simulink model "20240109_HVDCMMCInterconnection"  (R2023b)
settings: Solver=FixedStepDiscrete  StartTime=0.0  StopTime=2  FixedStep=Ts_Power  RelTol=1e-4  EnableMultiTasking=on
PreLoadFcn:
  | HVDCMMCInterconnectionParam
StartFcn:
  | tic
StopFcn:
  | toc
values from neighbouring files (symbols this model uses):
  C_PM = 1.758e-3    (= 0.001758)    [HVDCMMCInterconnectionParam.m]
  Cg = 50e-9    (= 5e-08)    [HVDCMMCInterconnectionParam.m]
  D_R = 0.001    [HVDCMMCInterconnectionParam.m]
  D_Rs = 1e8    (= 100000000)    [HVDCMMCInterconnectionParam.m]
  D_Vf = 0    [HVDCMMCInterconnectionParam.m]
  Fnom = 50    [HVDCMMCInterconnectionParam.m]
  HRM = 2    [HVDCMMCInterconnectionParam.m]
  Ki_Ireg = 6    [HVDCMMCInterconnectionParam.m]
  Ki_Preg = 1.0    (= 1)    [HVDCMMCInterconnectionParam.m]
  Ki_Qreg = 1.0    (= 1)    [HVDCMMCInterconnectionParam.m]
  Ki_VDCreg = 100    [HVDCMMCInterconnectionParam.m]
  Kp_Ireg = 0.6    [HVDCMMCInterconnectionParam.m]
  Kp_Preg = 0.5/3    (= 0.166666666667)    [HVDCMMCInterconnectionParam.m]
  Kp_Qreg = 0.5/3    (= 0.166666666667)    [HVDCMMCInterconnectionParam.m]
  Kp_VDCreg = 4    [HVDCMMCInterconnectionParam.m]
  L_cable = 15e-3    (= 0.015)    [HVDCMMCInterconnectionParam.m]
  Larm = Larm_pu*(Zb_ac/(2*pi*Fnom))    [HVDCMMCInterconnectionParam.m]
  Lff = Larm_pu/2    (= 0.075)    [HVDCMMCInterconnectionParam.m]
  Limits_Ireg = [ 2.0  -2.0]    [HVDCMMCInterconnectionParam.m]
  Limits_Preg = [ 1.2, 0.8 ]    [HVDCMMCInterconnectionParam.m]
  Limits_Qreg = [ 0.25, -0.25 ]    [HVDCMMCInterconnectionParam.m]
  Limits_VDCreg = [ 2.0  -2.0]    [HVDCMMCInterconnectionParam.m]
  Lxfo = 0.12    [HVDCMMCInterconnectionParam.m]
  Nb_PM = 36    [HVDCMMCInterconnectionParam.m]
  Pnom = 1000e6    (= 1000000000)    [HVDCMMCInterconnectionParam.m]
  R_cable = 0.5    [HVDCMMCInterconnectionParam.m]
  R_startup = 400    [HVDCMMCInterconnectionParam.m]
  Rarm = Rarm_pu*Zb_ac    [HVDCMMCInterconnectionParam.m]
  Rff = Rarm_pu/2    (= 0.00075)    [HVDCMMCInterconnectionParam.m]
  Rg = 100    [HVDCMMCInterconnectionParam.m]
  Rxfo = 0.003    [HVDCMMCInterconnectionParam.m]
  Slope_Pref = 0.5    [HVDCMMCInterconnectionParam.m]
  Slope_Qref = 0.5    [HVDCMMCInterconnectionParam.m]
  Slope_Vdc_ref = Vnom_dc/5    (= 128000)    [HVDCMMCInterconnectionParam.m]
  Tbrk1_On = 0.1    [HVDCMMCInterconnectionParam.m]
  Tbrk2_On = 1.0    (= 1)    [HVDCMMCInterconnectionParam.m]
  Tdeblock = 1.5    [HVDCMMCInterconnectionParam.m]
  Tfault = 9999    [HVDCMMCInterconnectionParam.m]
  Ton_Converter2 = 4    [HVDCMMCInterconnectionParam.m]
  Ton_PQreg = 4    [HVDCMMCInterconnectionParam.m]
  Ton_VDCreg = 1.5    [HVDCMMCInterconnectionParam.m]
  Ts = Ts_Control    (= 4e-05)    [HVDCMMCInterconnectionParam.m]
  Ts_Control = 40e-6    (= 4e-05)    [HVDCMMCInterconnectionParam.m]
  Ts_Power = 20e-6    (= 2e-05)    [HVDCMMCInterconnectionParam.m]
  Vb_ac = sqrt(2/3)*Vnom_sec    [HVDCMMCInterconnectionParam.m]
  Vb_dc = Vnom_dc    (= 640000)    [HVDCMMCInterconnectionParam.m]
  Vc0_PM = 0    [HVDCMMCInterconnectionParam.m]
  Vnom_dc = 640e3    (= 640000)    [HVDCMMCInterconnectionParam.m]
  Vnom_prim = 400e3    (= 400000)    [HVDCMMCInterconnectionParam.m]
  Vnom_sec = 333e3    (= 333000)    [HVDCMMCInterconnectionParam.m]
  w = 2*pi*Fnom    (= 314.159265359)    [HVDCMMCInterconnectionParam.m]
undefined symbols (not defined in the file or in its folder): DiscIntNeverNeededParam, gcbh, Pcc, S, sps_AC, sps_ACDC2, sps_rtmsupport
libraries: simulink x48, spsControlledVoltageSourceLib x30, spsCurrentMeasurementLib x30, MMC_Lib x30, spsDiodeLib x20, spsSeriesRLCBranchLib x14, powerlib_extras x12, spsVoltageMeasurementLib x12, spsSecondOrderFilterLib x8, spsabctodq0Lib x8, spsGroundLib x7, spsMeanLib x4
(part 1 of 9)
settings Model: SimulationMode=accelerator  Creator=The MathWorks, Inc.  LastModifiedBy=rober
settings SolverCC: ConcurrentTasks=on  ZeroCrossAlgorithm=Adaptive  InsertRTBMode=Always
settings DataIOCC: SaveFormat=StructureWithTime  SaveOutput=off  SignalLogging=off  DSMLogging=off  SaveTime=off  ReturnWorkspaceOutputs=off
settings OptimizationCC: ReuseModelBlockBuffer=off  ExpressionDepthLimit=2147483647  LifeSpan=inf
settings DebuggingCC: UnderspecifiedInitializationDetection=Classic  MergeDetectMultiDrivingBlocksExec=none  SolverPrmCheckMsg=warning  FcnCallInpInsideContextMsg=warning  AllowSymbolicDim=off  StateNameClashWarn=warning  SFUnexpectedBacktrackingDiag=warning  SFNoUnconditionalDefaultTransitionDiag=warning  SFExecutionAtInitializationDiag=none  ArithmeticOperatorsInVariantConditions=warning
settings HardwareCC: ProdBitPerPointer=32  ProdBitPerSizeT=32  ProdBitPerPtrDiffT=32  ProdLargestAtomicFloat=None  ProdIntDivRoundTo=Undefined  ProdEndianess=Unspecified  ProdWordSize=32  ProdHWDeviceType=32-bit Generic
settings ModelReferenceCC: EnableRefExpFcnMdlSchedulingChecks=on  PropagateSignalLabelsOutOfModel=off
settings SFSimCC: SimUseLocalCustomCode=off  CustomCodeUndefinedFunction=UseInterfaceOnly
settings RTWCC: RTWUseLocalCustomCode=off
settings CodeAppCC: StateflowObjectComments=on
settings GRTTargetCC: CombineOutputUpdateFcns=off  GRTInterface=on
settings ConfigComp: CovMetricSettings=dw  CovSaveCumulativeToWorkspaceVar=on  CovSaveSingleToWorkspaceVar=on  CovExternalEMLEnable=off
settings SimscapeCC: SimscapeNormalizeSystem=off

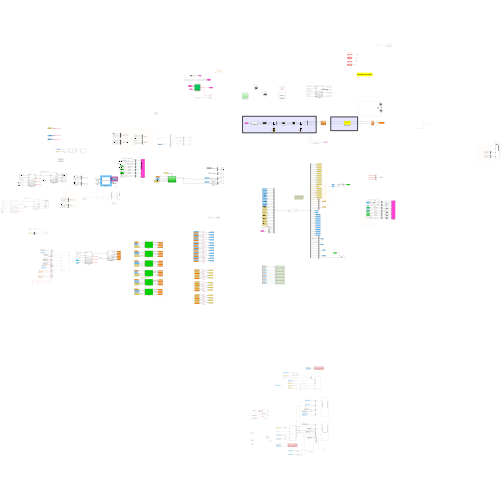
[thumbnail: Simulink's stored preview of the top-level diagram]
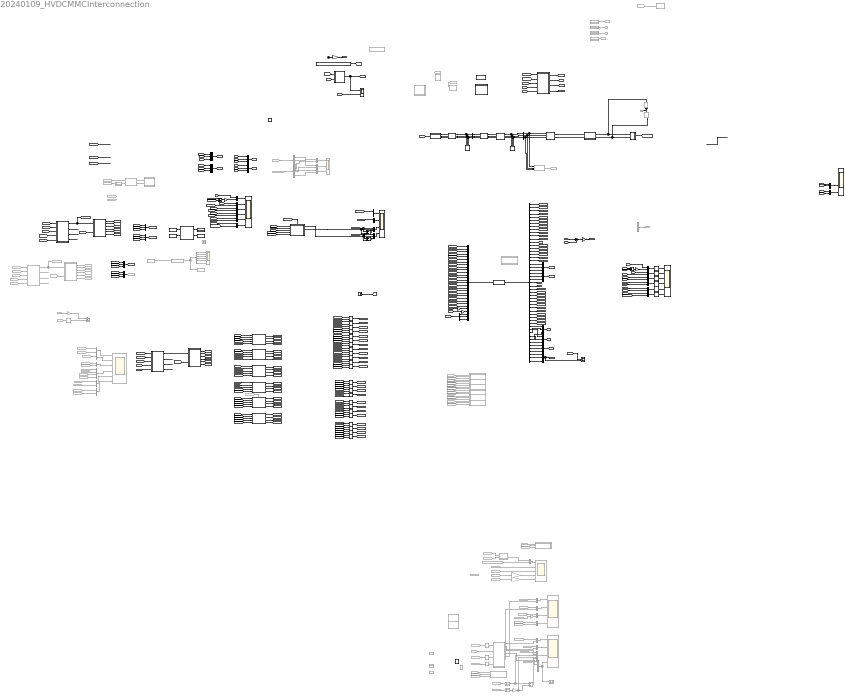
== system 20240109_HVDCMMCInterconnection ==
  note: HVDC-MMC Control System
  3ph SM1 : Subsystem  Commented=on
  3ph SM10 : Subsystem  Commented=on
  3ph SM11 : Subsystem  Commented=on
  3ph SM12 : Subsystem  Commented=on
  3ph SM13 : Subsystem  Commented=on
  3ph SM14 : Subsystem  Commented=on
  3ph SM2 : Subsystem  Commented=on
  3ph SM9 : Subsystem  Commented=on
  Add1 : Sum  Inputs=-+
  Add5 : Sum  Inputs=-+
  Brk1 : spsThreePhaseBreakerLib/Three-Phase Breaker  Commented=on  InitialState=open  SwitchA=on  SwitchB=on  SwitchC=on  SwitchTimes=0.1  External=on  BreakerResistance=0.001  SnubberResistance=1e6  SnubberCapacitance=inf  Measurements=Breaker voltages and currents
  Brk2 : spsThreePhaseBreakerLib/Three-Phase Breaker  Commented=on  InitialState=open  SwitchA=on  SwitchB=on  SwitchC=on  SwitchTimes=[30/60]*10000  External=on  BreakerResistance=0.01  SnubberResistance=1e6  SnubberCapacitance=inf  Measurements=Breaker voltages and currents
  COMPARE : Scope  NumInputPorts=6
  COMPARE1 : Scope  NumInputPorts=6
  Clock : Clock
  Constant3 : Constant  Value=complex( [[ 0 Vnom_prim*sqrt(2/3); 0 0; 0 0] zeros(3,HRM-1) ])
  Control : Subsystem
  Control1 : Subsystem
  Control2 : Subsystem
  Control3 : Subsystem  Commented=on
  Conv 2 : Subsystem
      settings: PortSchema="{\"entries\":[{\"content\":{\"sides\":[{\"content\":{\"connectorIds\":[\"LConn1\",\"LConn2\"]},\"type\":\"ConnectorPlacement.EquallySpacedRectSide\",\"uuid\":\"34e68c3c-08e2-4036-96f4-bd6ca1a4adc7\"},{\"content\":{\"connectorIds\":[\"In1\"],\"side\":\"RIGHT\"},\"type\":\"ConnectorPlacement.EquallySpacedRectSide\",\"uuid\":\"8026f2da-b291-4e86-8efa-4dfa5391ad34\"},{\"content\":{\"side\":\"TOP\"},\"type\":\"ConnectorPlacement.EquallySpacedRectSide\",\"uuid\":\"2a5049d1-3deb-4ece-8237-adb3b31cd77f\"}]},\"type\":\"ConnectorPlacement.EquallySpacedConnector\",\"uuid\":\"95075630-e580-4539-9cf3-c9c75bab0a7f\"}],\"packageUris\":[\"http://schema.mathworks.com/mf0/Connector/R2020b\"],\"version\":\"1.0\"}"
  DC & converter 2 : Subsystem
      mask Display: disp('DC circuit')
  DQn->ABC : MATLAB Function  TreatAsAtomicUnit=on  SystemSampleTime=Ts_Power  mask{N=HRM}
      mask prompts: N "Harmonic order:"
  Delay{,3,10..11} (4 alike) : Delay  Commented=on  DelayLength=1  SampleTime=Ts_Power
  Delay1 : Subsystem  Commented=on
  Delay2 : Delay  DelayLength=1  SampleTime=Ts_Power
  Delay5 : Subsystem  Commented=on
  Delay6 : Subsystem  Commented=on
  Delay7 : Subsystem  Commented=on
  Delay8 : Subsystem  Commented=on
  Delay9 : Subsystem  Commented=on
  Demux : Demux  Outputs=3
  Demux1 : Demux  Commented=on  Outputs=6
  Demux6 : Demux  Outputs=numel(sps_ACDC2.outputs)
  Demux7 : Demux  Commented=on  Outputs=3
  Demux8 : Demux  Commented=on  Outputs=3
  Discrete State-Space : DiscreteStateSpace  A=sps_ACDC2.Adiscrete  B=sps_ACDC2.Bdiscrete  C=sps_ACDC2.Cdiscrete  D=sps_ACDC2.Ddiscrete  InitialCondition=sps_ACDC2.x0  SampleTime=Ts_Power
  Discrete State-Space1 : Subsystem  Commented=on  SystemSampleTime=Ts_Power  mask{A=sps_ACDC2.A, B=sps_ACDC2.B, C=sps_ACDC2.C, D=sps_ACDC2.D, InitVec=sps_ACDC2.x0, dt=Ts_Power, DQSYM=off, N=HRM, Ws=w}
      mask prompts: InitVec "Initial condition:"; dt "Time step (s):"; N "Harmonic number:"; Ws "Angular frequency (1/rad):"
      mask init:
      | % I = eye(size(A,1));
      | % INVR = I/(I-A*dt/2);
      | % Ad1 = INVR*(I+A*dt/2);
      | % Bd1 = INVR*B*dt/2;
      | % Cd1 = C*Ad1;
      | % Dd11 = C*INVR*B*dt/2+D;
      | % Dd12 = C*INVR*B*dt/2;
      | 
      |     I = eye(size(A,1));
      |     INVR = I/(I-A*dt/2);
      |     Ad1 = INVR*(I+A*dt/2);
      |     Bd1 = INVR*B;
      |     Cd1 = C*INVR*dt;
      |     Dd1 = Cd1*B/2 + D;
      | 
      | DQSYM = get_param(gcb,'DQSYM');
      | 
      | comp = 0;
      | 
      | if(strcmp(DQSYM,'on'))
      | 
      | %Calculating the PNZ matrices
      | 
      |     a = -0.5+0.866i;
      |     a2 = -0.5-0.866i;
      |     Sas = [1,a,a2;1,a2,a;1,1,1]/3;
      | 
      |     arows = size(Ad1,1)/3; %signal size
      |     acols = size(Ad1,2)/3; %signal size
      | 
      |     brows = size(Bd1,1)/3; %signal size
      |     bcols = size(Bd1,2)/3; %signal size
      | 
      |     crows = size(Cd1,1)/3; %signal size
      |     ccols = size(Cd1,2)/3; %signal size
      | 
      |     d1rows = size(Dd1,1)/3; %signal size
      |     d1cols = size(Dd1,2)/3; %signal size
      | 
      |     %%%%%%%%%%%%%%%%%%%%%%% Check for inconsistencies  %%%%%%%%%%%%%%%%%%%%%%%
      | 
      |     szMatA = size(A,1);
      |     iL = eye(szMatA);
      |     szMatiL = size(iL,1);
      | 
      |     if(szMatiL ~= szMatA || size(A,1) ~= size(A,2) || size(iL,1) ~= size(iL,2))
      |         error('[Int_DQN_Mat/swFeedback] check matrix A size!');
      |     end
      | 
      |     if(arows ~= brows || acols ~= ccols || crows ~= d1rows || bcols ~= d1cols)
      |         error('[Int_DQN_Mat/Initialize] the sizes of the state-space matrices!');
      |     end
      | 
      |     %%%%%%%%%%%%%%%%%%%%%%%%%%%%%%%%%%%%%%%%%%%%%%%%%%%%%%%%%%%%%%%
      | 
      | 
      |     %%%%%%%%%%%%%%%%%%%%%%% A --> Bpnz %%%%%%%%%%%%%%%%%%%%%%%
      |     Adc = complex(zeros(3*arows,3*acols));
      | 
      |     for i = 1 : arows
      |         for j = 1 : acols
      |             Adc((1:3) + (i-1)*3,(1:3) + (j-1)*3) = Sas*Ad1((1:3) + (i-1)*3,(1:3) + (j-1)*3)/Sas;
      |             %Adc((1:3) + (i-1)*3,(1:3) + (j-1)*3) = diag(diag(real(Adc((1:3) + (i-1)*3,(1:3) + (j-1)*3))));
      |             %Adc((1:3) + (i-1)*3,(1:3) + (j-1)*3) = diag(diag((Adc((1:3) + (i-1)*3,(1:3) + (j-1)*3))));
      | 
      |         end
      |     end
      |     %%%%%%%%%%%%%%%%%%%%%%%%%%%%%%%%%%%%%%%%%%%%%%%%%%%%%%%%%%%%%%%
      | 
      |     %%%%%%%%%%%%%%%%%%%%%%% B --> Bpnz %%%%%%%%%%%%%%%%%%%%%%%
      | 
      |     Bdc = complex(zeros(3*brows,3*bcols));
      | 
      |     for i = 1 : brows
      |         for j = 1 : bcols
      |             Bdc((1:3) + (i-1)*3,(1:3) + (j-1)*3) = Sas*Bd1((1:3) + (i-1)*3,(1:3) + (j-1)*3)/Sas;
      |             %Bdc((1:3) + (i-1)*3,(1:3) + (j-1)*3) = diag(diag(real(Bdc((1:3) + (i-1)*3,(1:3) + (j-1)*3))));
      |             %Bdc((1:3) + (i-1)*3,(1:3) + (j-1)*3) = diag(diag((Bdc((1:3) + (i-1)*3,(1:3) + (j-1)*3))));
      | 
      |         end
      |     end
      |     %%%%%%%%%%%%%%%%%%%%%%%%%%%%%%%%%%%%%%%%%%%%%%%%%%%%%%%%%%%%%%%
      | 
      |     %%%%%%%%%%%%%%%%%%%%%%% C --> Cpnz %%%%%%%%%%%%%%%%%%%%%%%
      | 
      |     Cdc = complex(zeros(3*crows,3*ccols));
      | 
      |     for i = 1 : crows
      |         for j = 1 : ccols
      |             Cdc((1:3) + (i-1)*3,(1:3) + (j-1)*3) = Sas*Cd1((1:3) + (i-1)*3,(1:3) + (j-1)*3)/Sas;
      |             %Cdc((1:3) + (i-1)*3,(1:3) + (j-1)*3) = diag(diag(real(Cdc((1:3) + (i-1)*3,(1:3) + (j-1)*3))));
      |             %Cdc((1:3) + (i-1)*3,(1:3) + (j-1)*3) = diag(diag((Cdc((1:3) + (i-1)*3,(1:3) + (j-1)*3))));
      |         end
      |     end
      |     %%%%%%%%%%%%%%%%%%%%%%%%%%%%%%%%%%%%%%%%%%%%%%%%%%%%%%%%%%%%%%%
      | 
      |     
      |     %%%%%%%%%%%%%%%%%%%%%%% D1 --> Cpnz %%%%%%%%%%%%%%%%%%%%%%%
      | 
      |     Ddc = complex(zeros(3*d1rows,3*d1cols));
      | 
      |     for i = 1 : d1rows
      |         for j = 1 : d1cols
      |             Ddc((1:3) + (i-1)*3,(1:3) + (j-1)*3) = Sas*Dd1((1:3) + (i-1)*3,(1:3) + (j-1)*3)/Sas;
      |             %Ddc1((1:3) + (i-1)*3,(1:3) + (j-1)*3) = diag(diag(real(Ddc1((1:3) + (i-1)*3,(1:3) + (j-1)*3))));
      |             %Ddc((1:3) + (i-1)*3,(1:3) + (j-1)*3) = diag(diag((Ddc((1:3) + (i-1)*3,(1:3) + (j-1)*3))));
      |         end
      |     end
      |     %%%%%%%%%%%%%%%%%%%%%%%%%%%%%%%%%%%%%%%%%%%%%%%%%%%%%%%%%%%%%%%
      | 
      |     Adc(abs(Adc)<2*eps) = 0;
      |     Bdc(abs(Bdc)<2*eps) = 0;
      |     Cdc(abs(Cdc)<2*eps) = 0;
      |     Ddc(abs(Ddc)<2*eps) = 0;
      | 
      |     InitVec_c = complex(zeros(brows*3,N+1));
      | 
      | 
      |     if(~isempty(InitVec))
      |         if(mod(numel(InitVec),3)~=0) 
      |             warning('[SS_DQNc_Mat] InitVec with wrong size --> needs to be a multiple of 3!'); 
      | 
      |         else
      |             for k = 1 : numel(InitVec)/3
      |                 InitVec_c((k-1)*3+1:(k-1)*3+3,1) = Sas*InitVec((k-1)*3+1:(k-1)*3+3)*exp(+1i*Ws*dt);
      |             end
      |         end
      |     end
      | 
      |     InitVec = InitVec_c;
      | 
      | 
      |     Ad1 = Adc;
      |     Bd1 = Bdc;
      |     Cd1 = Cdc;
      |     Dd1 = Ddc;
      | 
      |     comp = -1i*Ws*dt;
      | 
      | end
      settings: MinAlgLoopOccurrences=on
      settings: LibrarySourceBlock=|
      | spsSynchronousMachineModel/Discrete robust/State Space Model/Discretize
      | BE or Tustin
      mask Callback DQSYM:
      | EMT = get_param(gcb,'DQSYM');
      | 
      | if(strcmp(EMT,'on'))
      |    set_param(gcb,'MaskVisibilities',{'on','on','on','on','on','on','on','on','on'});
      | else
      |    set_param(gcb,'MaskVisibilities',{'on','on','on','on','on','on','on','off','off'});
      | end
      mask Display: disp(['{\color{red}\bf\fontsize{12}x(t) = Ad*x(t-dt)+Bd*u(t)}',newline,'{\color{gray}\bf\fontsize{12}y(t) = Cd*x(t-dt)+Dd*u(t)}'], 'texmode','on');
  Discrete State-Space2 : DiscreteStateSpace  Commented=on  A=S.A  B=S.B  C=S.C  D=S.D  InitialCondition=S.x0  SampleTime=S.Ts
  Divide : Product  Inputs=**
  From : From  Commented=on  GotoTag=Uref_Ap  TagVisibility=global
  From1 : From  Commented=on  GotoTag=Uref_An  TagVisibility=global
  From{85,90,100,119,190,192} (6 alike) : From  Commented=on  GotoTag=Ap_Icap
  From101 : From  Commented=on  GotoTag=Bp_Icap
  From102 : From  Commented=on  GotoTag=Ap_Vin  TagVisibility=global
  From103 : From  Commented=on  GotoTag=Ap_Vbl  TagVisibility=global
  From106 : From  Commented=on  GotoTag=Bn_Ipos
  From107 : From  Commented=on  GotoTag=I_Ap_Db  TagVisibility=global
  From108 : From  Commented=on  GotoTag=Bn_Icap
  From11 : From  Commented=on  GotoTag=Q
  From{27,44,48,81,113} (5 alike) : From  Commented=on  GotoTag=I_Ap_Dt  TagVisibility=global
  From118 : From  Commented=on  GotoTag=I_Ap_Db  TagVisibility=global
  From{36..37,86,91,120,191} (6 alike) : From  Commented=on  GotoTag=Ap_Ipos
  From13 : From  Commented=on  GotoTag=Vsec  TagVisibility=global
  From131 : From  Commented=on  GotoTag=U_Bp_SM
  From14 : From  Commented=on  GotoTag=Vsec_ss
  From188 : From  Commented=on  GotoTag=I_Ap_Dt_ss
  From189 : From  Commented=on  GotoTag=I_Ap_Db_ss
  From193 : From  Commented=on  GotoTag=Ap_Vbl_ss
  From194 : From  Commented=on  GotoTag=Ap_Vin_ss
  From195 : From  Commented=on  GotoTag=Ap_Vin_EMT  TagVisibility=global
  From196 : From  Commented=on  GotoTag=Vdc_ss
  From197 : From  Commented=on  GotoTag=Vsec_ss
  From2 : From  Commented=on  GotoTag=P
  From21 : From  Commented=on  GotoTag=Brk2_On  TagVisibility=global
  From229 : From  Commented=on  GotoTag=Vdc_ref  TagVisibility=global
  From23 : From  Commented=on  GotoTag=Brk1_On  TagVisibility=global
  From230 : From  Commented=on  GotoTag=Qref  TagVisibility=global
  From231 : From  Commented=on  GotoTag=Blk  TagVisibility=global
  From232 : From  Commented=on  GotoTag=SF_Usec1
  From233 : From  Commented=on  GotoTag=SF_Isec1
  From234 : From  Commented=on  GotoTag=PQreg_On  TagVisibility=global
  From235 : From  Commented=on  GotoTag=Bp_Ipos
  From236 : From  Commented=on  GotoTag=Cp_Icap
  From239 : From  Commented=on  GotoTag=An_Ipos
  From240 : From  Commented=on  GotoTag=An_Icap
  From242 : From  Commented=on  GotoTag=Cn_Ipos
  From243 : From  Commented=on  GotoTag=Cn_Icap
  From244 : From  Commented=on  GotoTag=Cp_Ipos
  From245 : From  Commented=on  GotoTag=Uref_Ap_ss
  From246 : From  Commented=on  GotoTag=Uref_Bp_ss
  From247 : From  Commented=on  GotoTag=Uref_Cp_ss
  From248 : From  Commented=on  GotoTag=Uref_An_ss
  From249 : From  Commented=on  GotoTag=Uref_Bn_ss
  From250 : From  Commented=on  GotoTag=Uref_Cn_ss
  From28 : From  Commented=on  GotoTag=U_Ap_Dt
  From34 : From  Commented=on  GotoTag=Uref_Ap  TagVisibility=global
  From39 : From  Commented=on  GotoTag=U_Ap_Dt
  From4 : From  Commented=on  GotoTag=Vdc_kV
  From5 : From  Commented=on  GotoTag=V1rmsLL
  From6 : From  Commented=on  GotoTag=Vsec_ABC
  From69 : From  Commented=on  GotoTag=U_Ap_SM
  From7 : From  Commented=on  GotoTag=An_Ipos
  From73 : From  Commented=on  GotoTag=U_Ap_Dt
  From74 : From  Commented=on  GotoTag=Ap_Vbl_EMT  TagVisibility=global
  From9 : From  Commented=on  GotoTag=An_Icap
  From96 : From  Commented=on  GotoTag=Uref_Ap  TagVisibility=global
  From98 : From  Commented=on  GotoTag=I_Ap_Db
  From99 : From  Commented=on  GotoTag=I_Ap_Dt
  Gain : Gain  Gain=0.5
  Gain1 : Gain  Commented=on  Gain=-1
  Gain2 : Gain  Commented=on  Gain=D_Rs/(D_R+D_Rs)
  Gain3 : Gain  Commented=on  Gain=0.5
  Gain4 : Gain  Commented=on  Gain=1/Vb_dc
  Gain5 : Gain  Gain=2*pi*50
  Gain6 : Gain  Gain=0.5
  Gain7 : Gain  Commented=on  Gain=1/Vb_dc
  Gain8 : Gain
  Gain9 : Gain
  Gates : Subsystem
  Goto123 : Goto  Commented=on  GotoTag=SF_Isec1
  Goto124 : Goto  Commented=on  GotoTag=Uref_Bn_sf1  TagVisibility=global
  Goto125 : Goto  Commented=on  GotoTag=Uref_An_sf1  TagVisibility=global
  Goto126 : Goto  Commented=on  GotoTag=Uref_Cn_sf1  TagVisibility=global
  Goto127 : Goto  Commented=on  GotoTag=Uref_Bp_sf1  TagVisibility=global
  Goto128 : Goto  Commented=on  GotoTag=Uref_Ap_sf1  TagVisibility=global
  Goto129 : Goto  Commented=on  GotoTag=Uref_Cp_sf1  TagVisibility=global
  Goto130 : Goto  Commented=on  GotoTag=Uref_ABC_SF1
  Goto8 : Goto  Commented=on  GotoTag=Vsec_ss
  Ground2 : spsGroundLib/Ground  Commented=on  LConnTagsString=a
  I->pu1 : Gain  Gain=0.5  SaturateOnIntegerOverflow=on  OutDataTypeStr=Inherit: Same as input  ParamDataTypeStr=Inherit: Same as input
  Ld1 : spsThreePhaseSeriesRLCLoadLib/Three-Phase Series RLC Load  LConnTagsString=A|B|C  Configuration=Y (grounded)  NominalVoltage=Vnom_prim  Vabc=[1e3 1e3 1e3]  Vabcp=[1e3 1e3 1e3]  NominalFrequency=Fnom  UnbalancedPower=off  ActivePower=P_Ld1  InductivePower=0  CapacitivePower=0  Pabc=[10e3 9e3 11e3]  QLabc=[100 90 110]  QCabc=[100 90 110]  Pabcp=[10e3 9e3 11e3]  QLabcp=[100 90 110]  QCabcp=[100 90 110]  Measurements=None  LoadType=constant Z
  Ld2 : spsThreePhaseSeriesRLCLoadLib/Three-Phase Series RLC Load  LConnTagsString=A|B|C  Configuration=Y (grounded)  NominalVoltage=Vnom_sec  Vabc=[1e3 1e3 1e3]  Vabcp=[1e3 1e3 1e3]  NominalFrequency=Fnom  UnbalancedPower=off  ActivePower=500e3  InductivePower=0  CapacitivePower=0  Pabc=[10e3 9e3 11e3]  QLabc=[100 90 110]  QCabc=[100 90 110]  Pabcp=[10e3 9e3 11e3]  QLabcp=[100 90 110]  QCabcp=[100 90 110]  Measurements=None  LoadType=constant Z
  MATLAB Function : MATLAB Function  Commented=on  TreatAsAtomicUnit=on
  MATLAB Function1 : MATLAB Function  Commented=on  TreatAsAtomicUnit=on
  MATLAB Function2 : MATLAB Function  Commented=on  SystemSampleTime=Ts_Power  mask{Ts=Ts_Power, D_R=D_R, D_Rs=D_Rs, Nb_SM=Nb_PM, C=C_PM}
      mask prompts: Ts "Time step (s):"; D_R "Resistance Ron (Ohms):"; D_Rs "Snubber resistance Rs (Ohms):"; Nb_SM "Number of submodules:"; C "Submodule capacitance (F):"
      settings: MinAlgLoopOccurrences=on
  MMC : Subsystem
  Model : Subsystem  Commented=on  AncestorBlock=spsDiodeModel/Discrete  mask(DiscreteModel){}
  Model1 : Subsystem  Commented=on  AncestorBlock=spsDiodeModel/Discrete  mask(DiscreteModel){}
  Model2 : Subsystem  Commented=on  AncestorBlock=spsDiodeModel/Discrete  mask(DiscreteModel){}
  Mux{,1,3..6,10..11,16,18,22,44..49} (17 alike) : Mux  Inputs=3
  Mux{2,12..15,17,31,38..43,52..53} (15 alike) : Mux  Inputs=2
  Mux{9,19..20,24..28,32..37} (14 alike) : Mux  Commented=on  Inputs=2
  Mux21 : Mux  Commented=on
  Mux23 : Mux  Inputs=numel(sps_ACDC2.inputs)
  Mux29 : Mux  Commented=on  Inputs=5
  Mux30 : Mux  Commented=on  Inputs=5
  Mux7 : Mux  Commented=on  Inputs=3
  Mux8 : Mux  Commented=on  Inputs=3
  P (MW) : Display  Commented=on
      settings: Format=bank  Decimation=5000
  Q (Mvar) : Display  Commented=on
      settings: Format=bank  Decimation=5000
  RL Src : spsThreePhaseSeriesRLCBranchLib/Three-Phase Series RLC Branch  LConnTagsString=A|B|C  RConnTagsString=A|B|C  BranchType=RL  Resistance=0.8929  Inductance=16.58e-3  Capacitance=1e-6  Measurements=None
  R_startup : spsThreePhaseSeriesRLCBranchLib/Three-Phase Series RLC Branch  LConnTagsString=A|B|C  RConnTagsString=A|B|C  BranchType=R  Resistance=R_startup/50  Inductance=Vnom_prim^2 / Pcc / (2*pi*Fnom)  Capacitance=1e-6  Measurements=None
  Rate Transition{,1..5} (6 alike) : RateTransition
  SW{,1..23} (24 alike) : MMC_Lib/SW  SystemSampleTime=-1  SSRTWFcnClass=[]  VariantActivationTime=update diagram  AllowFlexibleInterface=on  Latency=0  AutoFrameSizeCalculation=off
  Scope : Scope  Commented=on  NumInputPorts=6
  Scope1 : Scope  NumInputPorts=2
  Scope10 : Scope  Commented=on  NumInputPorts=6
  Scope13 : Scope  NumInputPorts=4
  Scope2 : Scope  Commented=on  NumInputPorts=5
  Scope3 : Scope  Commented=on  NumInputPorts=4
  Scope4 : Scope  Commented=on  NumInputPorts=3
  Scope5 : Scope  Commented=on  NumInputPorts=4
  Scope6 : Scope  NumInputPorts=4
  Scope7 : Scope  Commented=on
  Scope8 : Scope  NumInputPorts=2
  Scope9 : Scope  Commented=on
  Scopes & Measurements : Subsystem  Commented=on
  Selector : Selector  Commented=on  InputPortWidth=3  IndexOptions=Index vector (dialog)  Indices=[1]  OutputSizes=1
  Sequencer : Subsystem
      mask Display: disp('Sequencer')
  Sources : Subsystem
  Sources1 : Subsystem  Commented=on
  State-Space : S-Function  FunctionName=sfun_spssw_discc  Parameters=S.Ts,S.A, S.B, S.C, S.D, S.x0, S.EnableUseOfTLC,S.SwitchResistance ,S.SwitchType, S.SwitchGateInitialValue, S.OutputsToResetToZero, S.TBEON,S.SaveMatrices,S.BufferSize  SFunctionDeploymentMode=off  EnableBusSupport=off
  Status : From  Commented=on  GotoTag=T43_3835_2986319703090  TagVisibility=global
      settings: CloseFcn=tagdialog Close
  Status1 : Subsystem
  Status_Bottom : From  Commented=on  GotoTag=T42_3768_2839018950081  TagVisibility=global
      settings: CloseFcn=tagdialog Close
  Status_Top : From  Commented=on  GotoTag=T43_3835_2986319703090  TagVisibility=global
      settings: CloseFcn=tagdialog Close
  Status_Top1 : From  Commented=on  GotoTag=T43_3835_2986319703090  TagVisibility=global
      settings: CloseFcn=tagdialog Close
  Step : Step  Time=2  SampleTime=Ts_Power
  Subsystem : Subsystem  AncestorBlock=MMC_Lib/Subsystem
      settings: PortSchema="{\"entries\":[{\"content\":{\"sides\":[{\"content\":{\"connectorIds\":[\"In1\",\"In2\",\"In3\",\"In4\",\"In5\"]},\"type\":\"ConnectorPlacement.EquallySpacedRectSide\",\"uuid\":\"b7415a3a-059a-466d-a519-c19f63b714af\"},{\"content\":{\"connectorIds\":[\"Out1\",\"Out2\",\"Out3\",\"Out4\"],\"side\":\"RIGHT\"},\"type\":\"ConnectorPlacement.EquallySpacedRectSide\",\"uuid\":\"984beb61-c57c-4d2a-959b-3a61047ea667\"},{\"content\":{\"connectorIds\":[\"In6\"],\"side\":\"TOP\"},\"type\":\"ConnectorPlacement.EquallySpacedRectSide\",\"uuid\":\"184f05c1-6fe5-4e4c-8e83-c1431acf6740\"}]},\"type\":\"ConnectorPlacement.EquallySpacedConnector\",\"uuid\":\"ac4715c0-a7f3-4877-877b-fb86a389a1b7\"}],\"packageUris\":[\"http://schema.mathworks.com/mf0/Connector/R2020b\"],\"version\":\"1.0\"}"
  Subsystem{1..6} (6 alike) : MMC_Lib/Subsystem  SystemSampleTime=-1  SSRTWFcnClass=[]  VariantActivationTime=update diagram  AllowFlexibleInterface=on  Latency=0  AutoFrameSizeCalculation=off
      settings: PortSchema="{\"entries\":[{\"content\":{\"sides\":[{\"content\":{\"connectorIds\":[\"In1\",\"In2\",\"In3\",\"In4\",\"In5\"]},\"type\":\"ConnectorPlacement.EquallySpacedRectSide\",\"uuid\":\"b7415a3a-059a-466d-a519-c19f63b714af\"},{\"content\":{\"connectorIds\":[\"Out1\",\"Out2\",\"Out3\",\"Out4\"],\"side\":\"RIGHT\"},\"type\":\"ConnectorPlacement.EquallySpacedRectSide\",\"uuid\":\"984beb61-c57c-4d2a-959b-3a61047ea667\"},{\"content\":{\"connectorIds\":[\"In6\"],\"side\":\"TOP\"},\"type\":\"ConnectorPlacement.EquallySpacedRectSide\",\"uuid\":\"184f05c1-6fe5-4e4c-8e83-c1431acf6740\"}]},\"type\":\"ConnectorPlacement.EquallySpacedConnector\",\"uuid\":\"ac4715c0-a7f3-4877-877b-fb86a389a1b7\"}],\"packageUris\":[\"http://schema.mathworks.com/mf0/Connector/R2020b\"],\"version\":\"1.0\"}"
  Subtract : Sum  Commented=on  Inputs=+-
  Subtract1 : Sum  Commented=on  Inputs=+-
  Subtract2 : Sum  Inputs=+-
  Subtract3 : Sum  Inputs=+-
  Sum2 : Sum  Inputs=|+-
  Tr1 : spsThreePhaseTransformerTwoWindingsLib/Three-Phase Transformer (Two Windings)  Winding1Connection=Yg  Winding2Connection=Yg  CoreType=Three single-phase transformers  SetSaturation=off  Hysteresis=off  DataFile='hysteresis'  SetInitialFlux=off  Measurements=None  UNITS=pu  NominalPower=[ Pnom , Fnom ]  Winding1="[ Vnom_prim , Rxfo/2,  Lxfo/2 ]"  Winding2="[ Vnom_sec , Rxfo/2,  Lxfo/2 ]"  Rm=1000  Lm=1000  L0=0.5  Saturation=[ 0,0 ; 0.0024,1.2 ; 1.0,1.52 ]  InitialFluxes=[ 0.8 , -0.8 , 0.7 ]  BreakLoop=off  DiscreteSolver=Trapezoidal iterative  DataType=off  TransfoNumber=1
  USW_Bottom : From  Commented=on  GotoTag=T43_3867_2942891286788  TagVisibility=global
  USW_Bottom1 : From  Commented=on  GotoTag=T43_3867_2942891286788  TagVisibility=global
  USW_Bottom3 : From  Commented=on  GotoTag=T43_3867_2942891286788  TagVisibility=global
  USW_Top{1..4} (4 alike) : From  Commented=on  GotoTag=T44_3934_3096165412659  TagVisibility=global
  Uref2m1 : Subsystem  Commented=on
  Uref2m2 : Subsystem
  Uref2m3 : Subsystem
  Uref2m4 : Subsystem  Commented=on
  V1 (kV rms LL) : Display  Commented=on
      settings: Format=bank  Decimation=5000
  VS Conv2b : spsControlledVoltageSourceLib/Controlled Voltage Source  Commented=on  Initialize=on  Source_Type=AC  Amplitude=0  Phase=0  Frequency=0  Measurements=None
  VS Conv2t : spsControlledVoltageSourceLib/Controlled Voltage Source  Commented=on  Initialize=on  Source_Type=AC  Amplitude=0  Phase=0  Frequency=0  Measurements=None
  Vdc (kV) : Display  Commented=on
      settings: Format=bank  Decimation=5000
  Voltage source : Subsystem
  Voltage source1 : Subsystem  Commented=on
  Yout : Subsystem
  Yout1 : Subsystem  Commented=on
  param : Subsystem  Commented=on
      settings: OpenFcn=open('HVDCMMCInterconnectionParam')
      mask Display: disp('Double-click to open\nparameters file')
  powergui : spspowerguiLib/powergui  Priority=1  SimulationMode=Discrete  SampleTime=Ts_Power  frequency=60  Iterations=50  frequencyindice=0  Pbase=100e6  ErrMax=1e-4  UnitsV=kV  UnitsW=MW  buscounter=0  FunctionMessages=off  echomessages=off  EnableUseOfTLC=off  CurrentSourceSwitches=off  DisableSnubberDevices=off  DisableRonSwitches=off  DisableVfSwitches=off  DisplayEquations=off  AutomaticDiscreteSolvers=off  SolverType=Tustin/Backward Euler (TBE)  Interpol=off  ExternalGateDelay=off  methode=off  Ts=10  x0status=blocks  SPID=off  SwTol=0  HookPort=off  NonlinearTolerance=1e-4  nMaxIteration=100  ContinueOnMaxIteration=off  RestoreLinks=warning  ResistiveCurrentMeasurement=off  Frange=[0:2:500]  Ylog=off  Xlog=on  ShowGrid=off  save=off  variable=ZData  structure=VIprim  ZoomFFT=on  StartTime=0.15  cycles=2  DisplayStyle=1  fundamental=50  FreqAxis=on  MaxFrequency=1000  frequencyindicesteady=1  RmsSteady=1  display=off
  prim : spsThreePhaseVIMeasurementLib/Three-Phase V-I Measurement  VoltageMeasurement=phase-to-ground  SetLabelV=on  LabelV=Vprim  Vpu=off  VpuLL=off  CurrentMeasurement=yes  SetLabelI=on  LabelI=Iprim  Ipu=off  Pbase=100e6  Vbase=500e3  OutputType=Complex  PhasorSimulation=off  PSBequivalent=0
  sec : spsThreePhaseVIMeasurementLib/Three-Phase V-I Measurement  VoltageMeasurement=phase-to-ground  SetLabelV=on  LabelV=Vsec  Vpu=off  VpuLL=off  CurrentMeasurement=yes  SetLabelI=on  LabelI=Isec  Ipu=off  Pbase=100e6  Vbase=500e3  OutputType=Complex  PhasorSimulation=off  PSBequivalent=0
  tag scope: Id_ss=global, SW=global, Uref_ABC=global, Uref_An_sf=global, Uref_Ap_sf=global, Uref_Bn_sf=global, Uref_Bp_sf=global, Uref_Cn_sf=global, Uref_Cp_sf=global, Vsrc_ABC=global, m1_dq=global, meas1=global, wt0=global, wt=global
  wires:
  From2/1 -> P (MW)/1
  From4/1 -> Vdc (kV)/1
  From5/1 -> V1 (kV rms LL)/1
  From11/1 -> Q (Mvar)/1
  From/1 -> Uref2m1/1(In1)
  [PQreg_On] -> Control/1(PQreg_ON)
  [Vdc_ref] -> Control/2(Vdc_ref)
  [Qref] -> Control/3(Qref)
  [Vsec] -> Control/4(Vsec)
  [Isec] -> Control/5(Isec)
  Control/1(Uref) -> [Uref_ABC]
  Control/2(Meas) -> [meas1]
  Control/3(m1_dq) -> [m1_dq]
  Control/4(wt) -> [wt]
  [Vsrc_ABC] -> Voltage source/1(In1)
  [wt0] -> DQn->ABC/2(tho)  "theta"
  [VSRC_C] -> DQn->ABC/1(Xdcpnz_c)  "[N+1,18 (6+6+6)]"
  [Vsec] -> Scope8/2
  DQn->ABC/1(Xabc) -> Scope8/1, [Vsrc_ABC]  "Mac_EMT"
  Constant3/1 -> [VSRC_C]
  Gain5/1 -> [wt0]
  Clock/1 -> Gain5/1
  From6/1 -> Voltage source1/1(In1)
  From21/1 -> Brk2/1
  [Isec_SS] -> Mux2/2
  Mux3/1 -> Scope6/3
  [Iprim] -> Mux3/1
  Mux2/1 -> Scope6/4
  [Isec] -> Mux2/1
  [Iprim_SS] -> Mux3/2
  Mux12/1 -> COMPARE/1
  [Idc1] -> Mux12/1  "Idc_EMT"
  [SF_Idc1p] -> Add5/1
  [SF_Idc1n] -> Add5/2
  Add5/1 -> Gain/1
  Gain/1 -> Mux12/2  "Idc_ss"
  [Vsec] -> Mux13/1  "Vsec_EMT"
  [SF_Usec] -> Mux13/2  "Vsec_ss"
  [Isec] -> Mux14/1  "Isec_EMT"
  [SF_Isec] -> Mux14/2  "Isec_ss"
  Mux15/1 -> COMPARE/2
  [SF_DC_Vdc1] -> Mux15/2  "Vdc_ss"
  [Vdc1] -> Mux15/1  "Vdc_EMT"
  Mux13/1 -> COMPARE/3
  Mux14/1 -> COMPARE/4
  [Id_ss] -> Mux17/2  "Idiff_ss"
  [Id_abc] -> Mux17/1  "Idiff_EMT"
  Mux17/1 -> COMPARE/5
  [I_Ap] -> Mux/1
  [I_Bp] -> Mux/2
  [I_Cp] -> Mux/3
  Mux26/1 -> Scope4/3
  Demux8/1 -> Mux27/1  "Target"
  Demux8/3 -> Mux26/1  "Target"
  Demux7/3 -> Mux26/2
  Demux7/1 -> Mux27/2
  Demux7/2 -> Mux25/2
  Demux8/2 -> Mux25/1  "Target"
  Mux27/1 -> Scope4/1
  Mux25/1 -> Scope4/2
  From13/1 -> Demux8/1
  From14/1 -> Demux7/1
  [V12_Ap] -> Mux11/1  "Ap"
  [V12_Cp] -> Mux11/3
  [V12_Bp] -> Mux11/2
  Mux11/1 -> [Vp_EMT]
  [Ip_ss] -> Sum2/1
  [In_ss] -> Sum2/2
  I->pu1/1 -> [Id_ss]
  Sum2/1 -> I->pu1/1  "Idiff"
  [I_Cm] -> Mux16/3
  [I_Am] -> Mux16/1
  [I_Bm] -> Mux16/2
  Mux/1 -> [Ip_EMT]
  Mux16/1 -> [Im_EMT]
  Mux10/1 -> [Vm_EMT]
  [V12_Am] -> Mux10/1  "Am"
  [V12_Cm] -> Mux10/3  "Am"
  [V12_Bm] -> Mux10/2  "Am"
  Mux31/1 -> COMPARE/6
  [Uref_ABC] -> Mux31/1
  [Uref_ABC_SF] -> Mux31/2
  Mux23/1 -> Discrete State-Space/1
  Discrete State-Space/1 -> Demux6/1
  [I_Cp_Db] -> Mux23/11
  [I_Cn_Db] -> Mux23/9
  [I_Cn_Dt] -> Mux23/10
  [I_Cp_Dt] -> Mux23/12
  [Bn_Vbl] -> Mux23/17
  [Bp_Vbl] -> Mux23/19
  [Bp_Vin] -> Mux23/20
  [Bn_Vin] -> Mux23/18
  [Cp_Vin] -> Mux23/24
  [Cn_Vbl] -> Mux23/21
  [Cp_Vbl] -> Mux23/23
  [Cn_Vin] -> Mux23/22
  [Vdc2b] -> Gain8/1
  [Vdc2t] -> Gain9/1
  Demux/1 -> Mux23/27
  Demux/2 -> Mux23/28
  Demux/3 -> Mux23/29
  [Vsrc_ABC] -> Demux/1
  Demux6/49 -> Mux18/1
  Demux6/50 -> Mux18/2
  Demux6/51 -> Mux18/3
  Demux6/46 -> Mux22/1
  Demux6/47 -> Mux22/2
  Demux6/48 -> Mux22/3
  Mux22/1 -> [Iprim_ss]
  Mux18/1 -> Scope1/2, [Isec_ss]
  [Isec] -> Scope1/1
  Mux7/1 -> Goto8/1
  ? -> Mux7/1
  ? -> Mux7/3
  ? -> Mux7/2
  Demux6/1 -> [U_An_Db]
  Demux6/2 -> [U_An_Dt]
  Demux6/3 -> [U_Ap_Db]
  Demux6/4 -> [U_Ap_Dt]
  Demux6/5 -> [U_Bn_Db]
  Demux6/6 -> [U_Bn_Dt]
  Demux6/7 -> [U_Bp_Db]
  Demux6/8 -> [U_Bp_Dt]
  Demux6/9 -> [U_Cn_Db]
  Demux6/10 -> [U_Cn_Dt]
  Demux6/11 -> [U_Cp_Db]
  Demux6/12 -> [U_Cp_Dt]
  Demux6/13 -> [Vdc_ss]
  Demux6/14 -> [U_An_SM]
  Demux6/15 -> [U_Ap_SM]
  Demux6/16 -> [U_Bn_SM]
  Demux6/17 -> [U_Bp_SM]
  Demux6/18 -> [U_Cn_SM]
  Demux6/19 -> [U_Cp_SM]
  Demux6/21 -> Mux1/2
  Demux6/22 -> Mux1/3
  Demux6/20 -> Mux1/1
  Mux1/1 -> [Vprim_ss]
  Mux4/1 -> [Vsec_ss]
  Demux6/25 -> Mux4/3
  Demux6/23 -> Mux4/1
  Demux6/24 -> Mux4/2
  Demux6/27 -> [Idc1p_ss]
  Demux6/26 -> [Idc1n_ss]
  Demux6/28 -> [An_Icap]
  Demux6/29 -> [An_Ipos]
  Demux6/30 -> [Ap_Icap]
  Demux6/31 -> [Ap_Ipos]
  Demux6/32 -> [Bn_Icap]
  Demux6/33 -> [Bn_Ipos]
  Demux6/34 -> [Bp_Icap]
  Demux6/35 -> [Bp_Ipos]
  Demux6/38 -> [Cp_Icap]
  Demux6/39 -> [Cp_Ipos]
  Demux6/36 -> [Cn_Icap]
  Demux6/37 -> [Cn_Ipos]
  Demux6/40 -> Mux6/1
  Demux6/43 -> Mux5/2
  Demux6/41 -> Mux5/1
  Demux6/42 -> Mux6/2
  Demux6/45 -> Mux5/3
  Demux6/44 -> Mux6/3
  Mux5/1 -> [Ip_ss]
  Mux6/1 -> [In_ss]
  From1/1 -> 3ph SM1/1(Uref_An)
  From7/1 -> 3ph SM1/2(An_Ipos)
  From9/1 -> 3ph SM1/3(An_Icap)
  MATLAB Function1/1(usw) -> Model/1(Uswitch)  "Uswitch"
  MATLAB Function1/2(status) -> Model/2(status)  "Status"
  From27/1 -> Scope2/2  "U_Ap_Dt"
  From28/1 -> Scope2/3  "U_Ap_Dt"
  From102/1 -> Gain4/1  "Ap_Vin"
  From103/1 -> Gain7/1  "Ap_Vbl"
  Status/1 -> Mux9/2  "Status"
  Gain4/1 -> Scope2/4  "Ap_Vin"
  Gain7/1 -> Scope2/5  "Ap_Vbl"
  Mux9/1 -> Scope2/1
  MATLAB Function/2(status) -> Mux9/1
  From44/1 -> MATLAB Function/1(Id)  "U_Ap_Dt"
  From39/1 -> MATLAB Function/2(Vd)  "U_Ap_Dt"
  From81/1 -> MATLAB Function1/1(Id)  "U_Ap_Dt"
  From73/1 -> Delay1/1(In1)  "U_Ap_Dt"
  [Converter2_On] -> Conv 2/1(On)
  Delay1/1(Out1) -> MATLAB Function1/2(Vd)
  [U_Ap_SM] -> ?  "U_Ap_SM"
  [Ap_Icap] -> ?  "Ap_Ipos"
  [Ap_Ipos] -> ?  "Ap_Icap"
  ? -> Model2/1(Uswitch)  "USW_Bottom_fcn"
  ? -> Model2/2(status)  "Status_Bottom_Fcn"
  ? -> Model1/1(Uswitch)  "USW_Top"
  ? -> Model1/2(status)  "Status_Top"
  From85/1 -> 3ph SM2/3(Ap_Icap)
  From34/1 -> 3ph SM2/1(Uref_Ap)
  From36/1 -> 3ph SM2/2(Ap_Ipos)
  From91/1 -> Delay10/1  "Ap_Icap"
  From69/1 -> Delay3/1  "U_Ap_SM"
  From90/1 -> Delay11/1  "Ap_Ipos"
  Delay11/1 -> MATLAB Function2/4(Ic)
  Delay10/1 -> MATLAB Function2/3(Ip)
  Delay3/1 -> MATLAB Function2/1(Usm)
  MATLAB Function2/1(UDt) -> Mux24/2  "USW_Top_fcn"
  USW_Top2/1 -> Mux24/1  "USW_Top"
  Mux24/1 -> Scope3/1
  Mux28/1 -> Scope3/2
  USW_Bottom/1 -> Mux28/1  "USW_Bottom"
  MATLAB Function2/3(UDb) -> Mux28/2  "USW_Bottom_fcn"
  Mux29/1 -> Scope3/3
  Status_Top/1 -> Mux29/1  "Status_Top"
  MATLAB Function2/2(Stt) -> Mux29/2  "Status_Top"
  Mux30/1 -> Scope3/4, Scope7/1
  Status_Bottom/1 -> Mux30/1  "Status_Bottom"
  MATLAB Function2/4(Stb) -> Mux30/2  "Status_Bottom_Fcn"
  Mux35/1 -> Scope5/4
  Mux33/1 -> Scope5/2
  Mux34/1 -> Scope5/3
  Mux32/1 -> Scope5/1
  From118/1 -> Mux35/2
  MATLAB Function2/6(IDb) -> Mux33/2  "Db_fcn"
  MATLAB Function2/5(IDt) -> Mux32/2  "Dt_fcn"
  From48/1 -> Mux32/1  "I_Ap_Dt"
  From107/1 -> Mux33/1  "I_Ap_Db"
  USW_Top3/1 -> Mux34/1  "USW_Top"
  Gain1/1 -> Mux34/2
  USW_Bottom1/1 -> Gain1/1  "USW_Bottom"
  From113/1 -> Mux35/1  "I_Ap_Dt"
  From119/1 -> Delay8/1(In1)  "Ap_Ipos"
  Delay9/1(Out1) -> Mux29/3, Subtract/1  "Ipos"
  From120/1 -> Delay9/1(In1)  "Ap_Icap"
  Delay8/1(Out1) -> Gain2/1  "Icap"
  Gain2/1 -> Mux29/4, Subtract/2
  Subtract/1 -> Mux29/5  "Ib"
  [Ap_Vbl] -> Mux23/15
  [Ap_Vin] -> Mux23/16
  From96/1 -> MATLAB Function2/2(Uref)
  [I_Ap_Dt_EMT] -> SW3/1
  [I_Ap_Db_EMT] -> SW2/1
  Control1/2(Meas) -> ?
  [Vsec] -> Control1/4(Vsec)
  [Qref] -> Control1/3(Qref)
  Control1/3(m1_dq) -> ?
  Control1/4(wt) -> ?
  [PQreg_On] -> Control1/1(PQreg_ON)
  [Isec] -> Control1/5(Isec)
  [Vdc_ref] -> Control1/2(Vdc_ref)
  [Blk] -> Uref2m2/2(Block)
  Control1/1(Uref) -> Uref2m2/1(Uref_ABC)
  Uref2m2/1(Uref_Ap) -> [Uref_Ap_ss]
  Subsystem1/2 -> [I_Ap_Dt_ss]  "Status_Top"
  Subsystem1/1 -> [I_Ap_Db_ss]  "Status_Bottom"
  Subsystem1/4 -> [Ap_Vin_ss]
  Subsystem1/3 -> [Ap_Vbl_ss]
  [I_Ap_Db_ss] -> SW2/2
  [I_Ap_Dt_ss] -> SW3/2
  Uref2m2/2(Uref_Bp) -> [Uref_Bp_ss]
  Uref2m2/5(Uref_Bn) -> [Uref_Bn_ss]
  Uref2m2/6(Uref_Cn) -> [Uref_Cn_ss]
  Uref2m2/4(Uref_An) -> [Uref_An_ss]
  Uref2m2/3(Uref_Cp) -> [Uref_Cp_ss]
  Subsystem2/4 -> [Bp_Vin_ss]
  [Bp_Icap] -> Subsystem2/3
  Subsystem2/1 -> [I_Bp_Db_ss]  "Status_Bottom"
  Subsystem2/2 -> [I_Bp_Dt_ss]  "Status_Top"
  [U_Bp_Dt] -> Subsystem2/4  "U_Ap_SM"
  [Uref_Bp_ss] -> Subsystem2/1
  Subsystem2/3 -> [Bp_Vbl_ss]
  [I_An_Dt_EMT] -> SW1/1
  [I_An_Db_ss] -> SW/2
  [I_An_Db_EMT] -> SW/1
  [I_An_Dt_ss] -> SW1/2
  [I_Bp_Dt_EMT] -> SW7/1
  [I_Bp_Db_ss] -> SW6/2
  [I_Bp_Db_EMT] -> SW6/1
  [I_Bp_Dt_ss] -> SW7/2
  [I_Bn_Dt_EMT] -> SW5/1
  [I_Bn_Db_EMT] -> SW4/1
  [I_Bn_Db_ss] -> SW4/2
  [I_Bn_Dt_ss] -> SW5/2
  [I_Bn_Dt_ss] -> SW9/2
  [I_Cp_Db_EMT] -> SW10/1
  [I_Cp_Dt_EMT] -> SW11/1
  [I_Cn_Db_EMT] -> SW8/1
  [I_Cn_Dt_EMT] -> SW9/1
  [I_Cp_Db_ss] -> SW10/2
  [I_Cn_Db_ss] -> SW8/2
  [I_Cp_Dt_ss] -> SW11/2
  [I_Bn_Db] -> Mux23/5
  [I_Bn_Dt] -> Mux23/6
  [I_Bp_Db] -> Mux23/7
  [I_Bp_Dt] -> Mux23/8
  SW7/1 -> [I_Bp_Dt]
  SW6/1 -> [I_Bp_Db]
  SW5/1 -> [I_Bn_Dt]
  SW4/1 -> [I_Bn_Db]
  SW/1 -> [I_An_Db]
  SW1/1 -> [I_An_Dt]
  SW2/1 -> [I_Ap_Db]
  SW3/1 -> [I_Ap_Dt]
  [I_Ap_Dt] -> Mux23/4
  [I_Ap_Db] -> Mux23/3
  [I_An_Dt] -> Mux23/2
  [I_An_Db] -> Mux23/1
  Step/1 -> [SW]
  SW8/1 -> [I_Cn_Db]
  SW9/1 -> [I_Cn_Dt]
  SW10/1 -> [I_Cp_Db]
  SW11/1 -> [I_Cp_Dt]
  [An_Vbl] -> Mux23/13
  [An_Vin] -> Mux23/14
  Subsystem4/2 -> [I_An_Dt_ss]  "Status_Top"
  Subsystem4/1 -> [I_An_Db_ss]  "Status_Bottom"
  Subsystem4/4 -> [An_Vin_ss]
  Subsystem6/1 -> [I_Cn_Db_ss]  "Status_Bottom"
  Subsystem6/2 -> [I_Cn_Dt_ss]  "Status_Top"
  Subsystem4/3 -> [An_Vbl_ss]
  Subsystem6/3 -> [Cn_Vbl_ss]
  Subsystem5/3 -> [Bn_Vbl_ss]
  Subsystem5/2 -> [I_Bn_Dt_ss]  "Status_Top"
  Subsystem5/1 -> [I_Bn_Db_ss]  "Status_Bottom"
  Subsystem6/4 -> [Cn_Vin_ss]
  Subsystem5/4 -> [Bn_Vin_ss]
  [An_Vbl_EMT] -> SW12/1
  [An_Vin_EMT] -> SW13/1
  [Ap_Vbl_EMT] -> SW14/1
  [Ap_Vin_EMT] -> SW15/1
  [Ap_Vbl_ss] -> SW14/2
  [Ap_Vin_ss] -> SW15/2
  [An_Vin_ss] -> SW13/2
  [An_Vbl_ss] -> SW12/2
  SW12/1 -> [An_Vbl]
  SW13/1 -> [An_Vin]
  SW14/1 -> [Ap_Vbl]
  SW15/1 -> [Ap_Vin]
  SW17/1 -> [Bn_Vin]
  [Bn_Vbl_EMT] -> SW16/1
  [Bp_Vbl_ss] -> SW18/2
  [Bn_Vbl_ss] -> SW16/2
  SW18/1 -> [Bp_Vbl]
  [Bn_Vin_ss] -> SW17/2
  [Bp_Vbl_EMT] -> SW18/1
  SW16/1 -> [Bn_Vbl]
  [Bp_Vin_ss] -> SW19/2
  [Bn_Vin_EMT] -> SW17/1
  SW19/1 -> [Bp_Vin]
  [Bp_Vin_EMT] -> SW19/1
  [Cp_Vin_EMT] -> SW23/1
  SW23/1 -> [Cp_Vin]
  [Cn_Vin_EMT] -> SW21/1
  [Cp_Vin_ss] -> SW23/2
  [Cp_Vbl_EMT] -> SW22/1
  SW21/1 -> [Cn_Vin]
  SW22/1 -> [Cp_Vbl]
  [Cn_Vin_ss] -> SW21/2
  [Cp_Vbl_ss] -> SW22/2
  [Cn_Vbl_ss] -> SW20/2
  [Cn_Vbl_EMT] -> SW20/1
  SW20/1 -> [Cn_Vbl]
  From197/1 -> Selector/1
  From196/1 -> Gain3/1
  Selector/1 -> Subtract1/2
  Gain3/1 -> Subtract1/1
  Sources/1(u) -> State-Space/1
  Gates/1(gates) -> State-Space/2
  State-Space/1 -> Yout/1(v,i)
  State-Space/2 -> Status1/1(status)
  Mux40/1 -> Rate Transition3/1
  Mux39/1 -> Rate Transition2/1
  Gain6/1 -> Mux38/2  "Idc_ss"
  [Vsec_ss] -> Mux39/2  "Vsec_ss"
  [Vdc_ss] -> Mux41/2  "Vdc_ss"
  [Uref_ABC_ss] -> Mux43/2
  Mux43/1 -> Rate Transition5/1
  [Uref_ABC] -> Mux43/1
  Mux42/1 -> Rate Transition4/1
  [Vdc1] -> Mux41/1  "Vdc_EMT"
  [Idc1n_ss] -> Add1/2
  Mux38/1 -> Rate Transition/1
  [Id_ss] -> Mux42/2  "Idiff_ss"
  [Idc1p_ss] -> Add1/1
  [Id_abc] -> Mux42/1  "Idiff_EMT"
  [Vsec] -> Mux39/1  "Vsec_EMT"
  [Isec_ss] -> Mux40/2  "Isec_ss"
  [Isec] -> Mux40/1  "Isec_EMT"
  Add1/1 -> Gain6/1
  Mux41/1 -> Rate Transition1/1
  [Idc1] -> Mux38/1  "Idc_EMT"
  [SF_Usec_a] -> Mux44/1
  [SF_Usec_b] -> Mux44/2
  [SF_Usec_c] -> Mux44/3
  Mux44/1 -> [SF_Usec]
  [SF_Isec_a] -> Mux45/1
  Mux45/1 -> [SF_Isec]
  [SF_Isec_b] -> Mux45/2
  [SF_Isec_c] -> Mux45/3
  [SF_Usec] -> Control2/4(Vsec)
  Control2/2(Meas) -> ?
  [Blk] -> Uref2m3/2(Block)
  [SF_Isec] -> Control2/5(Isec)
  Control2/3(m1_dq) -> ?
  [PQreg_On] -> Control2/1(PQreg_ON)
  Control2/4(wt) -> ?
  [Vdc_ref] -> Control2/2(Vdc_ref)
  [Qref] -> Control2/3(Qref)
  Control2/1(Uref) -> [Uref_ABC_SF], Uref2m3/1(Uref_ABC)
  Uref2m3/6(Uref_Cn) -> [Uref_Cn_sf]
  Uref2m3/4(Uref_An) -> [Uref_An_sf]
  Uref2m3/3(Uref_Cp) -> [Uref_Cp_sf]
  Uref2m3/1(Uref_Ap) -> [Uref_Ap_sf]
  Uref2m3/5(Uref_Bn) -> [Uref_Bn_sf]
  Uref2m3/2(Uref_Bp) -> [Uref_Bp_sf]
  Sources1/1(u) -> Discrete State-Space2/1
  Discrete State-Space2/1 -> Yout1/1(v,i), Demux1/1
  Mux46/1 -> [SF_Usec1]
  [SF_Isec_c1] -> Mux47/3
  [SF_Isec_b1] -> Mux47/2
  [SF_Isec_a1] -> Mux47/1
  Mux47/1 -> Goto123/1
  [SF_Usec_a1] -> Mux46/1
  [SF_Usec_b1] -> Mux46/2
  [SF_Usec_c1] -> Mux46/3
  Control3/1(Uref) -> Goto130/1, Uref2m4/1(Uref_ABC)
  From230/1 -> Control3/3(Qref)
  From229/1 -> Control3/2(Vdc_ref)
  Uref2m4/4(Uref_An) -> Goto125/1
  Uref2m4/3(Uref_Cp) -> Goto129/1
  Uref2m4/5(Uref_Bn) -> Goto124/1
  Uref2m4/2(Uref_Bp) -> Goto127/1
  Control3/4(wt) -> ?
  From234/1 -> Control3/1(PQreg_ON)
  From231/1 -> Uref2m4/2(Block)
  From232/1 -> Control3/4(Vsec)
  From233/1 -> Control3/5(Isec)
  Control3/3(m1_dq) -> ?
  Uref2m4/6(Uref_Cn) -> Goto126/1
  Uref2m4/1(Uref_Ap) -> Goto128/1
  Control3/2(Meas) -> ?
  Gain8/1 -> Mux23/25
  Gain9/1 -> Mux23/26
  Demux1/1 -> Scope10/1
  Demux1/2 -> Scope10/2
  Demux1/3 -> Scope10/3
  Demux1/4 -> Scope10/4
  Demux1/5 -> Scope10/5
  Demux1/6 -> Scope10/6
  [T43_3835_2986319703090] -> Mux52/1  "Status_Top"
  Mux52/1 -> Scope13/1
  [T42_3768_2839018950081] -> Mux53/1  "USW_Bottom"
  Mux53/1 -> Scope13/2
  [Ap_Ipos] -> Subsystem/2(Ipos)
  [U_Ap_Dt] -> Subsystem/4(UDt)
  [U_Ap_Db] -> Subsystem/5(UDb)
  [Ap_Icap] -> Subsystem/3(Icap)
  Mux48/1 -> Scope13/3
  Mux49/1 -> Scope13/4
  Subsystem/2(IDt) -> Mux48/2, Subtract3/2
  Subsystem/1(IDb) -> Subtract2/2, Mux49/2
  [I_Ap_Dt_EMT] -> Subtract3/1, Mux48/1
  [I_Ap_Db_EMT] -> Subtract2/1, Mux49/1
  Subtract2/1 -> Mux49/3
  Subtract3/1 -> Mux48/3
  From192/1 -> Mux21/4
  From191/1 -> Mux21/3
  ? -> Mux8/2  "USW_Top_ss"
  From188/1 -> Mux20/2  "I_Ap_Dt_ss"
  From99/1 -> Mux20/1  "I_Ap_Dt"
  USW_Top4/1 -> Mux8/1  "USW_Top"
  Mux21/1 -> Scope/4
  From74/1 -> Mux37/1  "Ap_Vbl"
  Mux37/1 -> Scope/6
  From195/1 -> Mux36/1  "Ap_Vin"
  From190/1 -> Mux8/3
  ? -> Mux19/2  "USW_Bottom_ss"
  From194/1 -> Mux36/2  "Ap_Vin_ss"
  From193/1 -> Mux37/2  "Ap_Vbl_ss"
  Mux36/1 -> Scope/5
  From189/1 -> Mux21/2  "I_Ap_Db_ss"
  Mux19/1 -> Scope/2
  USW_Bottom3/1 -> Mux19/1  "USW_Bottom"
  From98/1 -> Mux21/1  "I_Ap_Db"
  Mux8/1 -> Scope/1
  Mux20/1 -> Scope/3
  [Uref_Ap_ss] -> Subsystem/1(Uref)
  [U_Ap_SM] -> Subsystem/6(USM)  "U_Ap_SM"
  [Uref_Ap_ss] -> Subsystem1/1
  [Bp_Ipos] -> Subsystem2/2
  [U_Ap_Db] -> Subsystem1/5
  [U_Ap_Dt] -> Subsystem1/4
  [Ap_Icap] -> Subsystem1/2
  [Ap_Ipos] -> Subsystem1/3
  [U_Bp_Db] -> Subsystem2/5
  [U_Cp_Db] -> Subsystem3/5
  [U_Cp_Dt] -> Subsystem3/4  "U_Ap_SM"
  [Uref_Cp_ss] -> Subsystem3/1
  [Cp_Ipos] -> Subsystem3/2
  [Cp_Icap] -> Subsystem3/3
  Subsystem3/1 -> [I_Cp_Db_ss]  "Status_Bottom"
  Subsystem3/2 -> [I_Cp_Dt_ss]  "Status_Top"
  Subsystem3/3 -> [Cp_Vbl_ss]
  Subsystem3/4 -> [Cp_Vin_ss]
  [An_Ipos] -> Subsystem4/3
  [Uref_An_ss] -> Subsystem4/1
  From131/1 -> Subsystem5/6  "U_Ap_SM"
  [U_Bn_Db] -> Subsystem5/5
  [An_Icap] -> Subsystem4/2
  [U_Bn_Dt] -> Subsystem5/4  "U_Ap_SM"
  [Uref_Bn_ss] -> Subsystem5/1
  [Bn_Ipos] -> Subsystem5/2
  [Bn_Icap] -> Subsystem5/3
  [Cn_Icap] -> Subsystem6/3
  [Uref_Cn_ss] -> Subsystem6/1
  [U_Cn_Dt] -> Subsystem6/4  "U_Ap_SM"
  [U_Cn_Db] -> Subsystem6/5
  [Cn_Ipos] -> Subsystem6/2
  [U_An_Dt] -> Subsystem4/4
  [U_An_Db] -> Subsystem4/5
  From101/1 -> 3ph SM11/3(An_Icap)
  From86/1 -> 3ph SM10/2(An_Ipos)
  From100/1 -> 3ph SM10/3(An_Icap)
  From240/1 -> 3ph SM9/3(An_Icap)
  From236/1 -> 3ph SM13/3(An_Icap)
  From242/1 -> 3ph SM14/2(An_Ipos)
  From247/1 -> 3ph SM13/1(Uref_An)
  From244/1 -> 3ph SM13/2(An_Ipos)
  From249/1 -> 3ph SM12/1(Uref_An)
  From246/1 -> 3ph SM11/1(Uref_An)
  From245/1 -> 3ph SM10/1(Uref_An)
  From106/1 -> 3ph SM12/2(An_Ipos)
  From250/1 -> 3ph SM14/1(Uref_An)
  From108/1 -> 3ph SM12/3(An_Icap)
  From235/1 -> 3ph SM11/2(An_Ipos)
  From243/1 -> 3ph SM14/3(An_Icap)
  From239/1 -> 3ph SM9/2(An_Ipos)
  From248/1 -> 3ph SM9/1(Uref_An)
  Rate Transition/1 -> COMPARE1/1
  Rate Transition1/1 -> COMPARE1/2
  Rate Transition2/1 -> COMPARE1/3
  Rate Transition3/1 -> COMPARE1/4
  Rate Transition4/1 -> COMPARE1/5
  Rate Transition5/1 -> COMPARE1/6
  connections:
  Ld1/LConn1 -- RL Src/RConn1 -- prim/RConn1
  Ld1/LConn2 -- RL Src/RConn2 -- prim/RConn2
  Ld1/LConn3 -- RL Src/RConn3 -- prim/RConn3
  sec/RConn1 -- Ld2/LConn1 -- Tr1/RConn1
  sec/RConn2 -- Ld2/LConn2 -- Tr1/RConn2
  Ld2/LConn3 -- sec/RConn3 -- Tr1/RConn3
  prim/LConn1 -- R_startup/LConn1
  prim/LConn2 -- R_startup/LConn2
  prim/LConn3 -- R_startup/LConn3
  R_startup/RConn1 -- Tr1/LConn1
  R_startup/RConn2 -- Tr1/LConn2
  R_startup/RConn3 -- Tr1/LConn3
  Voltage source/RConn3 -- RL Src/LConn3
  Voltage source/RConn2 -- RL Src/LConn2
  Voltage source/RConn1 -- RL Src/LConn1
  MMC/RConn1 -- DC & converter 2/LConn1
  MMC/LConn1 -- Voltage source1/RConn1 -- sec/LConn1
  MMC/RConn2 -- DC & converter 2/LConn2
  MMC/LConn2 -- Voltage source1/RConn2 -- sec/LConn2
  MMC/LConn3 -- Voltage source1/RConn3 -- sec/LConn3
  ?
  VS Conv2t/LConn1 -- VS Conv2b/RConn1 -- Ground2/LConn1
  Conv 2/LConn1 -- VS Conv2t/RConn1 -- DC & converter 2/RConn1
  Conv 2/LConn2 -- VS Conv2b/LConn1 -- DC & converter 2/RConn2

== system 20240109_HVDCMMCInterconnection/3ph SM1 ==
  Uref_An : Inport
  An_Ipos : Inport  Port=2
  An_Icap : Inport  Port=3
  Demux : Demux  Outputs=2
  Demux2 : Demux  Outputs=2
  Discrete-Time Integrator1 : DiscreteIntegrator  IntegratorMethod=Integration: Trapezoidal  gainval=1  SampleTime=Ts_Power  UpperSaturationLimit=5000  LowerSaturationLimit=500  ICPrevOutput=DiscIntNeverNeededParam  ICPrevScaledInput=DiscIntNeverNeededParam
  Gain1 : Gain  Gain=Nb_PM
  Gain4 : Gain  Gain=1/(C_PM*Nb_PM)
  Gain5 : Gain  Gain=2
  Mux1 : Mux  Inputs=2
  Mux2 : Mux  Inputs=2
  Product3 : Product
  Product4 : Product
  Product7 : Product
  Sum3 : Sum  Inputs=1  InputSameDT=on  SaturateOnIntegerOverflow=on  OutDataTypeStr=Inherit: Same as first input
  Sum4 : Sum  Inputs=+-  InputSameDT=on  SaturateOnIntegerOverflow=on  OutDataTypeStr=Inherit: Same as first input
  Unit Delay5 : UnitDelay  SampleTime=Ts_Power  HasFrameUpgradeWarning=on
  Unit Delay6 : UnitDelay  SampleTime=Ts_Power  HasFrameUpgradeWarning=on
  Unit Delay7 : UnitDelay  SampleTime=Ts_Power  HasFrameUpgradeWarning=on
  An_Vbl : Outport
  An_Vin : Outport  Port=2
  wires:
  Gain5/1 -> Sum4/1
  Gain1/1 -> Demux2/1, Product3/1
  Mux2/1 -> Demux/1
  Demux/1 -> An_Vin/1
  Uref_An/1 -> Gain1/1
  Gain4/1 -> Discrete-Time Integrator1/1
  Mux1/1 -> Unit Delay7/1
  Demux2/2 -> Product7/1
  Unit Delay6/1 -> Gain5/1, Unit Delay5/1
  An_Icap/1 -> Mux1/2
  Demux2/1 -> Product4/1
  Discrete-Time Integrator1/1 -> Unit Delay6/1
  Sum4/1 -> Product7/2, Product4/2  "Vc"
  Unit Delay5/1 -> Sum4/2
  Sum3/1 -> Gain4/1
  Product3/1 -> Sum3/1
  Product4/1 -> Mux2/1  "Vin"
  Demux/2 -> An_Vbl/1
  Product7/1 -> Mux2/2  "Vbl"
  Unit Delay7/1 -> Product3/2
  An_Ipos/1 -> Mux1/1

== system 20240109_HVDCMMCInterconnection/3ph SM10 ==
  Uref_An : Inport
  An_Ipos : Inport  Port=2
  An_Icap : Inport  Port=3
  Demux : Demux  Outputs=2
  Demux2 : Demux  Outputs=2
  Discrete-Time Integrator1 : DiscreteIntegrator  IntegratorMethod=Integration: Trapezoidal  gainval=1  SampleTime=Ts_Power  UpperSaturationLimit=5000  LowerSaturationLimit=500  ICPrevOutput=DiscIntNeverNeededParam  ICPrevScaledInput=DiscIntNeverNeededParam
  Gain1 : Gain  Gain=Nb_PM
  Gain4 : Gain  Gain=1/(C_PM*Nb_PM)
  Gain5 : Gain  Gain=2
  Mux1 : Mux  Inputs=2
  Mux2 : Mux  Inputs=2
  Product3 : Product
  Product4 : Product
  Product7 : Product
  Sum3 : Sum  Inputs=1  InputSameDT=on  SaturateOnIntegerOverflow=on  OutDataTypeStr=Inherit: Same as first input
  Sum4 : Sum  Inputs=+-  InputSameDT=on  SaturateOnIntegerOverflow=on  OutDataTypeStr=Inherit: Same as first input
  Unit Delay5 : UnitDelay  SampleTime=Ts_Power  HasFrameUpgradeWarning=on
  Unit Delay6 : UnitDelay  SampleTime=Ts_Power  HasFrameUpgradeWarning=on
  Unit Delay7 : UnitDelay  SampleTime=Ts_Power  HasFrameUpgradeWarning=on
  An_Vbl : Outport
  An_Vin : Outport  Port=2
  wires:
  Gain5/1 -> Sum4/1
  Gain1/1 -> Demux2/1, Product3/1
  Mux2/1 -> Demux/1
  Demux/1 -> An_Vin/1
  Uref_An/1 -> Gain1/1
  Gain4/1 -> Discrete-Time Integrator1/1
  Mux1/1 -> Unit Delay7/1
  Demux2/2 -> Product7/1
  Unit Delay6/1 -> Gain5/1, Unit Delay5/1
  An_Icap/1 -> Mux1/2
  Demux2/1 -> Product4/1
  Discrete-Time Integrator1/1 -> Unit Delay6/1
  Sum4/1 -> Product7/2, Product4/2  "Vc"
  Unit Delay5/1 -> Sum4/2
  Sum3/1 -> Gain4/1
  Product3/1 -> Sum3/1
  Product4/1 -> Mux2/1  "Vin"
  Demux/2 -> An_Vbl/1
  Product7/1 -> Mux2/2  "Vbl"
  Unit Delay7/1 -> Product3/2
  An_Ipos/1 -> Mux1/1
